simulink model "UKF_Simple"  (Simulink 7.4)
settings: Solver=ode45  StartTime=0.0  StopTime=6000.0  RelTol=1e-3
libraries: aausat3_lib x9
settings Model: Creator=KFJensen  LastModifiedBy=KF Jensen
settings DataIOCC: LimitDataPoints=off
settings OptimizationCC: InlineParams=on  SimCompilerOptimization=On
settings DebuggingCC: SignalInfNanChecking=error  IntegerOverflowMsg=error  ParameterUnderflowMsg=error  AssertControl=DisableAll  StrictBusMsg=None
settings HardwareCC: ProdHWDeviceType=Generic->Unspecified (assume 32-bit Generic)

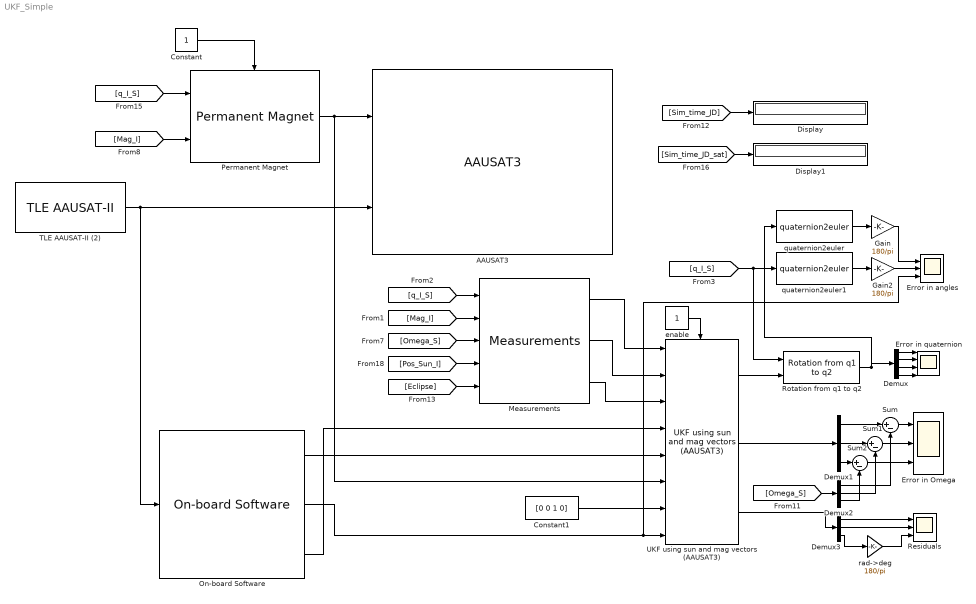
== system UKF_Simple ==
  AAUSAT3 : aausat3_lib/AAUSAT3  SystemSampleTime=-1  r_com_s=[0.049073,0.048909,0.041691]  sat_temp_start=293.15  mass_sc=0.957820  Dim=[0.1,0.1,0.11]  inertia_c=[0.0017466,0.0020972,0.0021268]  init_jd=2455153.1954318+0.035  q_s_c=[-0.018775,0.71389,-0.0072618,0.69997]  q_init_I_S=[0 0 0 1]  w_init_s=[0.02,0.02,0.02]  Cd=2  rho=5e-14  solar_m_flux=4.5565e-6  solar_absorb_coeff=1.5  theta_e=65  refldata=load('lib/AlbedoToolbox-1.0/refl_data/2005/ga050101-051231')  redfac=1  Ts=1  enable_sensor_emulation=on  enable_env_disturbance=on
  Constant : Constant  OutDataType=fixdt(1, 16)  OutScaling=2^0
  Constant1 : Constant  Value=[0 0 1 0]  OutDataType=fixdt(1, 16)  OutScaling=2^0
  Demux : Demux
  Demux1 : Demux  Outputs=3
  Demux2 : Demux  Outputs=3
  Demux3 : Demux  Outputs=3
  Display : Display
  Display1 : Display
  Error in Omega : Scope  NumInputPorts=3
      settings: TimeRange=2000  YMin=-0.002~-0.00175~-0.0015  YMax=0.0025~0.00125~0.0025  SampleInput=on  SampleTime=1
  Error in angles : Scope  NumInputPorts=3
      settings: TimeRange=2000  YMin=-7~-200~0  YMax=4~200~1  SaveName=ScopeData2  SampleInput=on  SampleTime=1
  Error in quaternion : Scope  NumInputPorts=4
      settings: TimeRange=250  YMin=-0.5~-0.25~-1~-1  YMax=0.5~0.25~1~1.25  SampleInput=on  SampleTime=1
  Gain : Gain  Gain=180/pi  ParameterDataType=fixdt(1, 16)  ParameterScaling=2^0  OutDataType=fixdt(1, 16)  OutScaling=2^0
  Gain2 : Gain  Gain=180/pi  ParameterDataType=fixdt(1, 16)  ParameterScaling=2^0  OutDataType=fixdt(1, 16)  OutScaling=2^0
  Measurements : aausat3_lib/Sensor Emulation/Measurements  SystemSampleTime=-1  s_freq_mag=1  noise_mag=3  bias_mag=[0 0 0]  heading_mag=0  tilt_mag=0  s_freq_sun=1  noise_sun=3.33  bias_sun=[0 0]  nr_sample_sun=1  s_freq_gyro=1  noise_gyro=0.2  bias_gyro=[0 0 0]  heading_gyro=0  tilt_gyro=0
  On-board Software : aausat3_lib/On-board Software  SystemSampleTime=-1  init_jd=2455153.1954318+0.035  igrf_order=8  theta_e=65  Ts=1
  Permanent Magnet : aausat3_lib/Actuator Emulation/Permanent Magnet  SystemSampleTime=-1  mag_moment=0.0030
  Residuals : Scope  NumInputPorts=3
      settings: TimeRange=6000  YMin=-1.1~-1.1~-1  YMax=1.1~1.1~1  SaveName=ScopeData3  SampleInput=on  SampleTime=1
  Rotation from q1 to q2 : aausat3_lib/Math Utilities/Quaternion operations/Rotation from q1 to q2  SystemSampleTime=-1
  Sum : Sum  Inputs=|+-  OutDataType=fixdt(1, 16)  OutScaling=2^0
  Sum1 : Sum  Inputs=|+-  OutDataType=fixdt(1, 16)  OutScaling=2^0
  Sum2 : Sum  Inputs=|+-  OutDataType=fixdt(1, 16)  OutScaling=2^0
  TLE AAUSAT-II (2) : aausat3_lib/Orbit and Ephemeris/TLE AAUSAT-II  SystemSampleTime=-1  satname='AAUSAT-II'  JulianDay=09321.69542252  xndt2o=0.00000555  xndd6o=0.0  bstar=.76898e-4  xincl=97.9251  xnodeo=24.1597  eo=0.0014245  omegao=254.1774  xmo=105.7862  xno=14.81823818  ts=1
  UKF using sun and mag vectors (AAUSAT3) : aausat3_lib/ADS/UKF using sun and mag vectors (AAUSAT3)  SystemSampleTime=-1  f_sample=1
      link override UKF: MATLABFcn=UKFsimple
  enable : Constant  OutDataType=fixdt(1, 16)  OutScaling=2^0
  quaternion2euler : aausat3_lib/Math Utilities/Quaternion operations/quaternion2euler  SystemSampleTime=-1
  quaternion2euler1 : aausat3_lib/Math Utilities/Quaternion operations/quaternion2euler  SystemSampleTime=-1
  rad->deg : Gain  Gain=180/pi  ParameterDataType=fixdt(1, 16)  ParameterScaling=2^0  OutDataType=fixdt(1, 16)  OutScaling=2^0
  wires:
  Permanent Magnet/1 -> UKF using sun and mag vectors (AAUSAT3)/6, AAUSAT3/1
  TLE AAUSAT-II (2)/1 -> On-board Software/1, AAUSAT3/2
  [q_I_S] -> Permanent Magnet/1
  [Mag_I] -> Permanent Magnet/2
  Constant/1 -> Permanent Magnet/Enable
  [q_I_S] -> Measurements/1
  [Mag_I] -> Measurements/2
  [Omega_S] -> Measurements/3
  Measurements/1 -> UKF using sun and mag vectors (AAUSAT3)/1
  Measurements/2 -> UKF using sun and mag vectors (AAUSAT3)/2
  Measurements/3 -> UKF using sun and mag vectors (AAUSAT3)/3
  Constant1/1 -> UKF using sun and mag vectors (AAUSAT3)/7
  UKF using sun and mag vectors (AAUSAT3)/1 -> Rotation from q1 to q2/2
  [q_I_S] -> Rotation from q1 to q2/1, quaternion2euler1/1
  Demux/1 -> Error in quaternion/1
  Demux/2 -> Error in quaternion/2
  Demux/3 -> Error in quaternion/3
  Demux/4 -> Error in quaternion/4
  Rotation from q1 to q2/1 -> Demux/1, quaternion2euler/1
  [Omega_S] -> Demux2/1
  Demux1/3 -> Sum2/1
  Demux2/3 -> Sum2/2
  Demux2/2 -> Sum1/2
  Demux2/1 -> Sum/2
  Sum1/1 -> Error in Omega/2
  Sum2/1 -> Error in Omega/3
  Sum/1 -> Error in Omega/1
  [Sim_time_JD] -> Display/1
  Gain/1 -> Error in angles/1
  [Sim_time_JD_sat] -> Display1/1
  Gain2/1 -> Error in angles/2
  [Eclipse] -> Measurements/5
  [Pos_Sun_I] -> Measurements/4
  quaternion2euler1/1 -> Gain2/1
  quaternion2euler/1 -> Gain/1
  On-board Software/2 -> Error in angles/3, UKF using sun and mag vectors (AAUSAT3)/8
  On-board Software/3 -> UKF using sun and mag vectors (AAUSAT3)/4
  Demux1/1 -> Sum/1
  Demux1/2 -> Sum1/1
  UKF using sun and mag vectors (AAUSAT3)/2 -> Demux1/1
  UKF using sun and mag vectors (AAUSAT3)/3 -> Demux3/1
  Demux3/1 -> Residuals/1
  Demux3/2 -> Residuals/2
  rad->deg/1 -> Residuals/3
  Demux3/3 -> rad->deg/1
  On-board Software/1 -> UKF using sun and mag vectors (AAUSAT3)/5
  enable/1 -> UKF using sun and mag vectors (AAUSAT3)/Enable
